simulink library "engine_T2_lib"  (Simulink 7.2)
settings: Solver=ode45  SolverMode=SingleTasking  StartTime=0.0  StopTime=10.0  RelTol=1e-3
undefined symbols (not defined in the file or in its folder): engl_ang, engr_ang, LengON, LinearizeModeOn, RengON, TrimModeOn
libraries: aeroutilslib x4, engine_JetCatP70_lib x4, simulink x3, Cross_Product_3D_lib x2
settings Model: Creator=amurch  LastModifiedBy=E183308

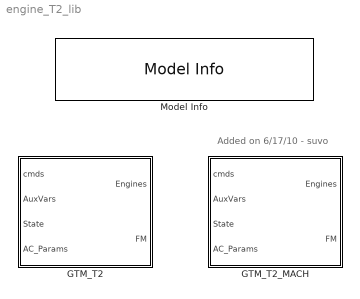
== system engine_T2_lib ==
  note: Added on 6/17/10 - suvo
  GTM_T2 : Subsystem
  GTM_T2_MACH : Subsystem
  Model Info : simulink/Model-Wide Utilities/Model Info  SystemSampleTime=-1  InitialBlockCM=None  BlockCM=None  Frame=on  DisplayStringWithTags=|  HorizontalTextAlignment=Center  LeftAlignmentValue=0.5  SourceBlockDiagram=engine_T2_lib  TagMaxNumber=20
      | GTM T2 Engine Library
      | 
      | Model Version: %<ModelVersion>
      | Last modifed by %<LastModifiedBy> on %<LastModificationDate>

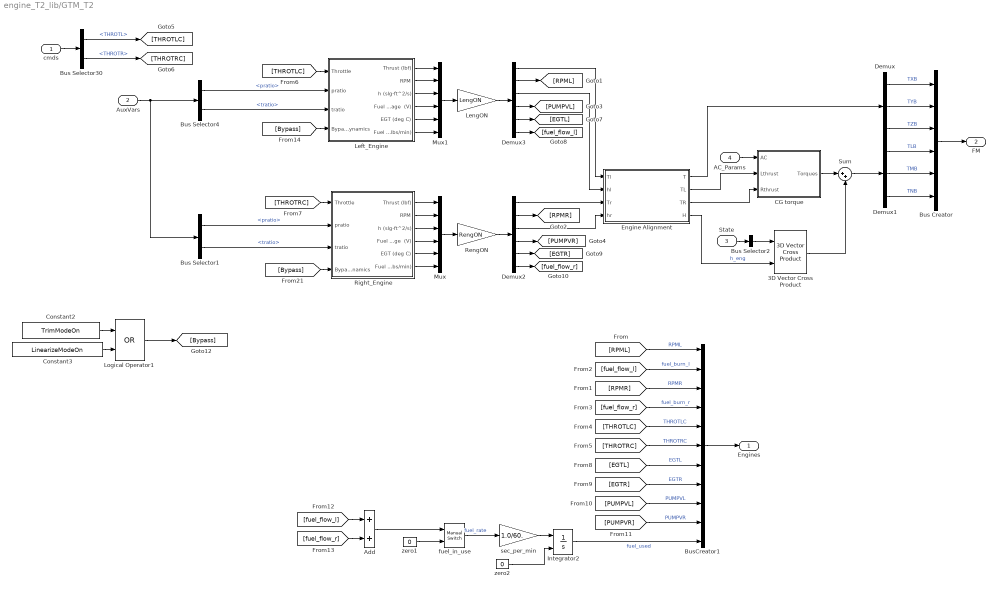
== system engine_T2_lib/GTM_T2 ==
  cmds : Inport  OutDataType=sfix(16)  OutScaling=2^0
  AuxVars : Inport  Port=2  OutDataType=sfix(16)  OutScaling=2^0
  State : Inport  Port=3  OutDataType=sfix(16)  OutScaling=2^0
  AC_Params : Inport  Port=4  OutDataType=sfix(16)  OutScaling=2^0
  3D Vector Cross Product : Cross_Product_3D_lib/3D Vector Cross Product  SystemSampleTime=-1
  Add : Sum  OutDataType=sfix(16)  OutScaling=2^-10
  Bus Creator : BusCreator  Inputs=6
  Bus Selector1 : BusSelector  OutputSignals=pratio,tratio
  Bus Selector2 : BusSelector  OutputSignals=pb,qb,rb  OutputAsBus=on
  Bus Selector30 : BusSelector  OutputSignals=THROTL,THROTR
  Bus Selector4 : BusSelector  OutputSignals=pratio,tratio
  BusCreator1 : BusCreator  Inputs=11
  CG torque : Subsystem
  Constant2 : Constant  Value=TrimModeOn  OutDataType=sfix(16)  OutScaling=2^0
  Constant3 : Constant  Value=LinearizeModeOn  OutDataType=sfix(16)  OutScaling=2^0
  Demux : Demux  Outputs=3
  Demux1 : Demux  Outputs=3
  Demux2 : Demux  Outputs=6
  Demux3 : Demux  Outputs=6
  Engine Alignment : Stateflow chart
  Integrator2 : Integrator  InitialConditionSource=external
  Left_Engine : Subsystem  BlockChoice=Jetcat P70
      settings: AttributesFormatString=%<BlockChoice>  TemplateBlock=enginelib/Engine Model  MemberBlocks=AMT-180,AMT-280,Blank,Jetcat P120SE,Jetcat P70
  LengON : Gain  Gain=LengON  ParameterDataType=sfix(16)  ParameterScaling=2^0  OutDataType=sfix(16)  OutScaling=2^0  SaturateOnIntegerOverflow=on  OutDataTypeStr=Inherit: Same as input  ParamDataTypeStr=Inherit: Same as input
  Logical Operator1 : Logic  Operator=OR  AllPortsSameDT=off  OutDataTypeMode=boolean  OutDataTypeStr=boolean
  Mux : Mux  Inputs=6
  Mux1 : Mux  Inputs=6
  RengON : Gain  Gain=RengON  ParameterDataType=sfix(16)  ParameterScaling=2^0  OutDataType=sfix(16)  OutScaling=2^0  SaturateOnIntegerOverflow=on  OutDataTypeStr=Inherit: Same as input  ParamDataTypeStr=Inherit: Same as input
  Right_Engine : Subsystem  BlockChoice=Jetcat P70
      settings: AttributesFormatString=%<BlockChoice>  TemplateBlock=enginelib/Engine Model  MemberBlocks=AMT-180,AMT-280,Blank,Jetcat P120SE,Jetcat P70
  Sum : Sum  Inputs=|++  OutDataType=sfix(16)  OutScaling=2^0
  fuel_in_use : simulink/Signal Routing/Manual Switch  SystemSampleTime=-1  sw=0  action=0  varsize=off
  sec_per_min : Gain  Gain=1.0/60.  ParameterDataType=sfix(16)  ParameterScaling=2^0  OutDataType=sfix(16)  OutScaling=2^0  SaturateOnIntegerOverflow=on  OutDataTypeStr=Inherit: Same as input  ParamDataTypeStr=Inherit: Same as input
  zero1 : Constant  Value=0  OutDataType=sfix(16)  OutScaling=2^0
  zero2 : Constant  Value=0  OutDataType=sfix(16)  OutScaling=2^0
  Engines : Outport  OutDataType=sfix(16)  OutScaling=2^0
  FM : Outport  Port=2  PortDimensions=6  OutDataType=sfix(16)  OutScaling=2^0
  wires:
  cmds/1 -> Bus Selector30/1
  Demux/2 -> Bus Creator/2  "TYB"
  State/1 -> Bus Selector2/1
  Bus Selector2/1 -> 3D Vector Cross Product/1
  Demux/3 -> Bus Creator/3  "TZB"
  Bus Selector1/1 -> Right_Engine/2(pratio)  "<pratio>"
  Bus Selector1/2 -> Right_Engine/3(tratio)  "<tratio>"
  AuxVars/1 -> Bus Selector1/1, Bus Selector4/1
  AC_Params/1 -> CG torque/1(AC)
  Bus Creator/1 -> FM/1
  Bus Selector30/1 -> [THROTLC]  "<THROTL>"
  Bus Selector30/2 -> [THROTRC]  "<THROTR>"
  [THROTLC] -> Left_Engine/1(Throttle)
  [THROTRC] -> Right_Engine/1(Throttle)
  [THROTRC] -> BusCreator1/6  "THROTRC"
  [THROTLC] -> BusCreator1/5  "THROTLC"
  [fuel_flow_r] -> BusCreator1/4  "fuel_burn_r"
  [fuel_flow_l] -> BusCreator1/2  "fuel_burn_l"
  [RPMR] -> BusCreator1/3  "RPMR"
  [RPML] -> BusCreator1/1  "RPML"
  BusCreator1/1 -> Engines/1
  [EGTL] -> BusCreator1/7  "EGTL"
  [EGTR] -> BusCreator1/8  "EGTR"
  [PUMPVL] -> BusCreator1/9  "PUMPVL"
  [PUMPVR] -> BusCreator1/10  "PUMPVR"
  sec_per_min/1 -> Integrator2/1
  fuel_in_use/1 -> sec_per_min/1  "fuel_rate"
  Integrator2/1 -> BusCreator1/11  "fuel_used"
  zero2/1 -> Integrator2/2
  [fuel_flow_l] -> Add/1
  [fuel_flow_r] -> Add/2
  zero1/1 -> fuel_in_use/2
  Add/1 -> fuel_in_use/1
  Bus Selector4/1 -> Left_Engine/2(pratio)  "<pratio>"
  Bus Selector4/2 -> Left_Engine/3(tratio)  "<tratio>"
  [Bypass] -> Left_Engine/4(BypassDynamics)
  [Bypass] -> Right_Engine/4(BypassDynamics)
  Demux/1 -> Bus Creator/1  "TXB"
  Engine Alignment/4(H) -> 3D Vector Cross Product/2  "h_eng"
  Engine Alignment/1(T) -> Demux/1
  Engine Alignment/2(TL) -> CG torque/2(Lthrust)
  Engine Alignment/3(TR) -> CG torque/3(Rthrust)
  CG torque/1(Torques) -> Sum/1
  3D Vector Cross Product/1 -> Sum/2
  Sum/1 -> Demux1/1
  Demux1/1 -> Bus Creator/4  "TLB"
  Demux1/2 -> Bus Creator/5  "TMB"
  Demux1/3 -> Bus Creator/6  "TNB"
  Right_Engine/1(Thrust (lbf)) -> Mux/1
  Right_Engine/2(RPM) -> Mux/2
  Right_Engine/3(h (slg-ft^2/s)) -> Mux/3
  Right_Engine/4(Fuel Pump Voltage  (V)) -> Mux/4
  Right_Engine/5(EGT (deg C)) -> Mux/5
  Right_Engine/6(Fuel Flow (lbs/min)) -> Mux/6
  Mux/1 -> RengON/1
  RengON/1 -> Demux2/1
  Demux2/1 -> Engine Alignment/3(Tr)
  Demux2/2 -> [RPMR]
  Demux2/3 -> Engine Alignment/4(hr)
  Demux2/4 -> [PUMPVR]
  Demux2/5 -> [EGTR]
  Demux2/6 -> [fuel_flow_r]
  Mux1/1 -> LengON/1
  LengON/1 -> Demux3/1
  Left_Engine/1(Thrust (lbf)) -> Mux1/1
  Left_Engine/2(RPM) -> Mux1/2
  Left_Engine/3(h (slg-ft^2/s)) -> Mux1/3
  Left_Engine/4(Fuel Pump Voltage  (V)) -> Mux1/4
  Left_Engine/5(EGT (deg C)) -> Mux1/5
  Left_Engine/6(Fuel Flow (lbs/min)) -> Mux1/6
  Demux3/1 -> Engine Alignment/1(Tl)
  Demux3/2 -> [RPML]
  Demux3/3 -> Engine Alignment/2(hl)
  Demux3/4 -> [PUMPVL]
  Demux3/5 -> [EGTL]
  Demux3/6 -> [fuel_flow_l]
  Constant3/1 -> Logical Operator1/2
  Constant2/1 -> Logical Operator1/1
  Logical Operator1/1 -> [Bypass]

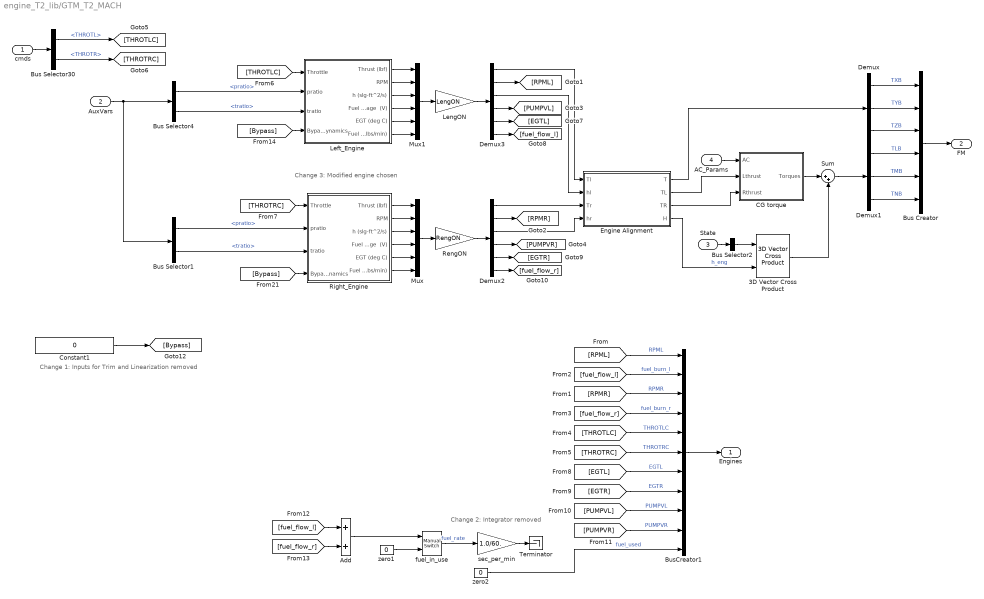
== system engine_T2_lib/GTM_T2_MACH ==
  note: Change 1: Inputs for Trim and Linearization removed
  note: Change 2: Integrator removed
  note: Change 3: Modified engine chosen
  cmds : Inport  OutDataType=sfix(16)  OutScaling=2^0
  AuxVars : Inport  Port=2  OutDataType=sfix(16)  OutScaling=2^0
  State : Inport  Port=3  OutDataType=sfix(16)  OutScaling=2^0
  AC_Params : Inport  Port=4  OutDataType=sfix(16)  OutScaling=2^0
  3D Vector Cross Product : Cross_Product_3D_lib/3D Vector Cross Product  SystemSampleTime=-1
  Add : Sum  OutDataType=sfix(16)  OutScaling=2^-10
  Bus Creator : BusCreator  Inputs=6
  Bus Selector1 : BusSelector  OutputSignals=pratio,tratio
  Bus Selector2 : BusSelector  OutputSignals=pb,qb,rb  OutputAsBus=on
  Bus Selector30 : BusSelector  OutputSignals=THROTL,THROTR
  Bus Selector4 : BusSelector  OutputSignals=pratio,tratio
  BusCreator1 : BusCreator  Inputs=11
  CG torque : Subsystem
  Constant1 : Constant  Value=0  OutDataType=sfix(16)  OutScaling=2^0
  Demux : Demux  Outputs=3
  Demux1 : Demux  Outputs=3
  Demux2 : Demux  Outputs=6
  Demux3 : Demux  Outputs=6
  Engine Alignment : Stateflow chart
  Left_Engine : Subsystem  BlockChoice=Jetcat P70_MACH
      settings: AttributesFormatString=%<BlockChoice>  TemplateBlock=enginelib/Engine Model  MemberBlocks=AMT-180,AMT-280,Blank,Jetcat P120SE,Jetcat P70,Jetcat P70_MACH
  LengON : Gain  Gain=LengON  ParameterDataType=sfix(16)  ParameterScaling=2^0  OutDataType=sfix(16)  OutScaling=2^0  SaturateOnIntegerOverflow=on  OutDataTypeStr=Inherit: Same as input  ParamDataTypeStr=Inherit: Same as input
  Mux : Mux  Inputs=6
  Mux1 : Mux  Inputs=6
  RengON : Gain  Gain=RengON  ParameterDataType=sfix(16)  ParameterScaling=2^0  OutDataType=sfix(16)  OutScaling=2^0  SaturateOnIntegerOverflow=on  OutDataTypeStr=Inherit: Same as input  ParamDataTypeStr=Inherit: Same as input
  Right_Engine : Subsystem  BlockChoice=Jetcat P70_MACH
      settings: AttributesFormatString=%<BlockChoice>  TemplateBlock=enginelib/Engine Model  MemberBlocks=AMT-180,AMT-280,Blank,Jetcat P120SE,Jetcat P70,Jetcat P70_MACH
  Sum : Sum  Inputs=|++  OutDataType=sfix(16)  OutScaling=2^0
  Terminator : Terminator
  fuel_in_use : simulink/Signal Routing/Manual Switch  SystemSampleTime=-1  sw=0  action=0  varsize=off
  sec_per_min : Gain  Gain=1.0/60.  ParameterDataType=sfix(16)  ParameterScaling=2^0  OutDataType=sfix(16)  OutScaling=2^0  SaturateOnIntegerOverflow=on  OutDataTypeStr=Inherit: Same as input  ParamDataTypeStr=Inherit: Same as input
  zero1 : Constant  Value=0  OutDataType=sfix(16)  OutScaling=2^0
  zero2 : Constant  Value=0  OutDataType=sfix(16)  OutScaling=2^0
  Engines : Outport  OutDataType=sfix(16)  OutScaling=2^0
  FM : Outport  Port=2  PortDimensions=6  OutDataType=sfix(16)  OutScaling=2^0
  wires:
  Constant1/1 -> [Bypass]
  Demux3/6 -> [fuel_flow_l]
  Demux3/5 -> [EGTL]
  Demux3/4 -> [PUMPVL]
  Demux3/3 -> Engine Alignment/2(hl)
  Demux3/2 -> [RPML]
  Demux3/1 -> Engine Alignment/1(Tl)
  Left_Engine/6(Fuel Flow (lbs/min)) -> Mux1/6
  Left_Engine/5(EGT (deg C)) -> Mux1/5
  Left_Engine/4(Fuel Pump Voltage  (V)) -> Mux1/4
  Left_Engine/3(h (slg-ft^2/s)) -> Mux1/3
  Left_Engine/2(RPM) -> Mux1/2
  Left_Engine/1(Thrust (lbf)) -> Mux1/1
  LengON/1 -> Demux3/1
  Mux1/1 -> LengON/1
  Demux2/6 -> [fuel_flow_r]
  Demux2/5 -> [EGTR]
  Demux2/4 -> [PUMPVR]
  Demux2/3 -> Engine Alignment/4(hr)
  Demux2/2 -> [RPMR]
  Demux2/1 -> Engine Alignment/3(Tr)
  RengON/1 -> Demux2/1
  Mux/1 -> RengON/1
  Right_Engine/6(Fuel Flow (lbs/min)) -> Mux/6
  Right_Engine/5(EGT (deg C)) -> Mux/5
  Right_Engine/4(Fuel Pump Voltage  (V)) -> Mux/4
  Right_Engine/3(h (slg-ft^2/s)) -> Mux/3
  Right_Engine/2(RPM) -> Mux/2
  Right_Engine/1(Thrust (lbf)) -> Mux/1
  Demux1/3 -> Bus Creator/6  "TNB"
  Demux1/2 -> Bus Creator/5  "TMB"
  Demux1/1 -> Bus Creator/4  "TLB"
  Sum/1 -> Demux1/1
  3D Vector Cross Product/1 -> Sum/2
  CG torque/1(Torques) -> Sum/1
  Engine Alignment/3(TR) -> CG torque/3(Rthrust)
  Engine Alignment/2(TL) -> CG torque/2(Lthrust)
  Engine Alignment/1(T) -> Demux/1
  Engine Alignment/4(H) -> 3D Vector Cross Product/2  "h_eng"
  Demux/1 -> Bus Creator/1  "TXB"
  [Bypass] -> Right_Engine/4(BypassDynamics)
  [Bypass] -> Left_Engine/4(BypassDynamics)
  Bus Selector4/2 -> Left_Engine/3(tratio)  "<tratio>"
  Bus Selector4/1 -> Left_Engine/2(pratio)  "<pratio>"
  Add/1 -> fuel_in_use/1
  zero1/1 -> fuel_in_use/2
  [fuel_flow_r] -> Add/2
  [fuel_flow_l] -> Add/1
  zero2/1 -> BusCreator1/11  "fuel_used"
  fuel_in_use/1 -> sec_per_min/1  "fuel_rate"
  sec_per_min/1 -> Terminator/1
  [PUMPVR] -> BusCreator1/10  "PUMPVR"
  [PUMPVL] -> BusCreator1/9  "PUMPVL"
  [EGTR] -> BusCreator1/8  "EGTR"
  [EGTL] -> BusCreator1/7  "EGTL"
  BusCreator1/1 -> Engines/1
  [RPML] -> BusCreator1/1  "RPML"
  [RPMR] -> BusCreator1/3  "RPMR"
  [fuel_flow_l] -> BusCreator1/2  "fuel_burn_l"
  [fuel_flow_r] -> BusCreator1/4  "fuel_burn_r"
  [THROTLC] -> BusCreator1/5  "THROTLC"
  [THROTRC] -> BusCreator1/6  "THROTRC"
  [THROTRC] -> Right_Engine/1(Throttle)
  [THROTLC] -> Left_Engine/1(Throttle)
  Bus Selector30/2 -> [THROTRC]  "<THROTR>"
  Bus Selector30/1 -> [THROTLC]  "<THROTL>"
  Bus Creator/1 -> FM/1
  AC_Params/1 -> CG torque/1(AC)
  AuxVars/1 -> Bus Selector4/1, Bus Selector1/1
  Bus Selector1/2 -> Right_Engine/3(tratio)  "<tratio>"
  Bus Selector1/1 -> Right_Engine/2(pratio)  "<pratio>"
  Demux/3 -> Bus Creator/3  "TZB"
  Bus Selector2/1 -> 3D Vector Cross Product/1
  State/1 -> Bus Selector2/1
  Demux/2 -> Bus Creator/2  "TYB"
  cmds/1 -> Bus Selector30/1

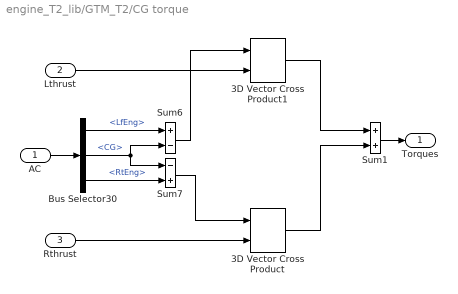
== system engine_T2_lib/GTM_T2/CG torque ==
  AC : Inport  OutDataType=sfix(16)  OutScaling=2^0
  Lthrust : Inport  Port=2  OutDataType=sfix(16)  OutScaling=2^0
  Rthrust : Inport  Port=3  OutDataType=sfix(16)  OutScaling=2^0
  3D Vector Cross Product : aeroutilslib/3D Vector Cross Product  SystemSampleTime=-1
  3D Vector Cross Product1 : aeroutilslib/3D Vector Cross Product  SystemSampleTime=-1
  Bus Selector30 : BusSelector  OutputSignals=LfEng,CG,RtEng
  Sum1 : Sum  OutDataType=sfix(16)  OutScaling=2^0  SaturateOnIntegerOverflow=on  InputSameDT=on  OutDataTypeStr=Inherit: Same as first input
  Sum6 : Sum  Inputs=+-  OutDataType=sfix(16)  OutScaling=2^0  SaturateOnIntegerOverflow=on  InputSameDT=on  OutDataTypeStr=Inherit: Same as first input
  Sum7 : Sum  Inputs=-+  OutDataType=sfix(16)  OutScaling=2^0  SaturateOnIntegerOverflow=on  InputSameDT=on  OutDataTypeStr=Inherit: Same as first input
  Torques : Outport  OutDataType=sfix(16)  OutScaling=2^0
  wires:
  AC/1 -> Bus Selector30/1
  Bus Selector30/2 -> Sum7/1, Sum6/2  "<CG>"
  Lthrust/1 -> 3D Vector Cross Product1/2
  Rthrust/1 -> 3D Vector Cross Product/2
  Sum7/1 -> 3D Vector Cross Product/1
  Sum6/1 -> 3D Vector Cross Product1/1
  3D Vector Cross Product1/1 -> Sum1/1
  3D Vector Cross Product/1 -> Sum1/2
  Sum1/1 -> Torques/1
  Bus Selector30/3 -> Sum7/2  "<RtEng>"
  Bus Selector30/1 -> Sum6/1  "<LfEng>"

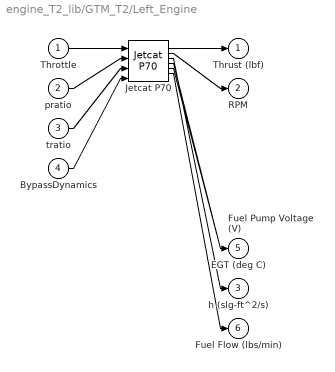
== system engine_T2_lib/GTM_T2/Left_Engine ==
  Throttle : Inport  OutDataType=sfix(16)  OutScaling=2^0
  pratio : Inport  Port=2  OutDataType=sfix(16)  OutScaling=2^0
  tratio : Inport  Port=3  OutDataType=sfix(16)  OutScaling=2^0
  BypassDynamics : Inport  Port=4  OutDataType=sfix(16)  OutScaling=2^0
  Jetcat P70 : engine_JetCatP70_lib/Jetcat P70  SystemSampleTime=-1
  Thrust (lbf) : Outport  OutDataType=sfix(16)  OutScaling=2^0
  RPM : Outport  Port=2  OutDataType=sfix(16)  OutScaling=2^0
  h (slg-ft^2/s) : Outport  Port=3  OutDataType=sfix(16)  OutScaling=2^0
  Fuel Pump Voltage  (V) : Outport  Port=4  OutDataType=sfix(16)  OutScaling=2^0
  EGT (deg C) : Outport  Port=5  OutDataType=sfix(16)  OutScaling=2^0
  Fuel Flow (lbs/min) : Outport  Port=6  OutDataType=sfix(16)  OutScaling=2^0
  wires:
  Throttle/1 -> Jetcat P70/1
  pratio/1 -> Jetcat P70/2
  tratio/1 -> Jetcat P70/3
  BypassDynamics/1 -> Jetcat P70/4
  Jetcat P70/1 -> Thrust (lbf)/1
  Jetcat P70/2 -> RPM/1
  Jetcat P70/3 -> h (slg-ft^2/s)/1
  Jetcat P70/4 -> Fuel Pump Voltage  (V)/1
  Jetcat P70/5 -> EGT (deg C)/1
  Jetcat P70/6 -> Fuel Flow (lbs/min)/1

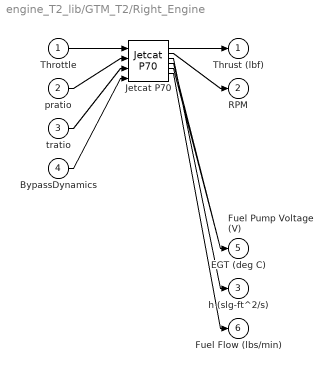
== system engine_T2_lib/GTM_T2/Right_Engine ==
  Throttle : Inport  OutDataType=sfix(16)  OutScaling=2^0
  pratio : Inport  Port=2  OutDataType=sfix(16)  OutScaling=2^0
  tratio : Inport  Port=3  OutDataType=sfix(16)  OutScaling=2^0
  BypassDynamics : Inport  Port=4  OutDataType=sfix(16)  OutScaling=2^0
  Jetcat P70 : engine_JetCatP70_lib/Jetcat P70  SystemSampleTime=-1
  Thrust (lbf) : Outport  OutDataType=sfix(16)  OutScaling=2^0
  RPM : Outport  Port=2  OutDataType=sfix(16)  OutScaling=2^0
  h (slg-ft^2/s) : Outport  Port=3  OutDataType=sfix(16)  OutScaling=2^0
  Fuel Pump Voltage  (V) : Outport  Port=4  OutDataType=sfix(16)  OutScaling=2^0
  EGT (deg C) : Outport  Port=5  OutDataType=sfix(16)  OutScaling=2^0
  Fuel Flow (lbs/min) : Outport  Port=6  OutDataType=sfix(16)  OutScaling=2^0
  wires:
  Throttle/1 -> Jetcat P70/1
  pratio/1 -> Jetcat P70/2
  tratio/1 -> Jetcat P70/3
  BypassDynamics/1 -> Jetcat P70/4
  Jetcat P70/1 -> Thrust (lbf)/1
  Jetcat P70/2 -> RPM/1
  Jetcat P70/3 -> h (slg-ft^2/s)/1
  Jetcat P70/4 -> Fuel Pump Voltage  (V)/1
  Jetcat P70/5 -> EGT (deg C)/1
  Jetcat P70/6 -> Fuel Flow (lbs/min)/1

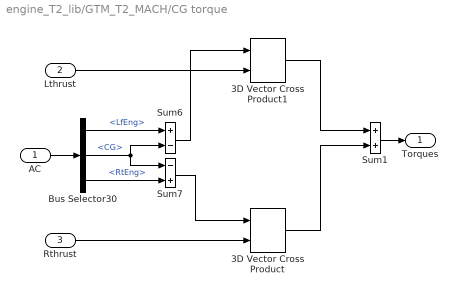
== system engine_T2_lib/GTM_T2_MACH/CG torque ==
  AC : Inport  OutDataType=sfix(16)  OutScaling=2^0
  Lthrust : Inport  Port=2  OutDataType=sfix(16)  OutScaling=2^0
  Rthrust : Inport  Port=3  OutDataType=sfix(16)  OutScaling=2^0
  3D Vector Cross Product : aeroutilslib/3D Vector Cross Product  SystemSampleTime=-1
  3D Vector Cross Product1 : aeroutilslib/3D Vector Cross Product  SystemSampleTime=-1
  Bus Selector30 : BusSelector  OutputSignals=LfEng,CG,RtEng
  Sum1 : Sum  OutDataType=sfix(16)  OutScaling=2^0  SaturateOnIntegerOverflow=on  InputSameDT=on  OutDataTypeStr=Inherit: Same as first input
  Sum6 : Sum  Inputs=+-  OutDataType=sfix(16)  OutScaling=2^0  SaturateOnIntegerOverflow=on  InputSameDT=on  OutDataTypeStr=Inherit: Same as first input
  Sum7 : Sum  Inputs=-+  OutDataType=sfix(16)  OutScaling=2^0  SaturateOnIntegerOverflow=on  InputSameDT=on  OutDataTypeStr=Inherit: Same as first input
  Torques : Outport  OutDataType=sfix(16)  OutScaling=2^0
  wires:
  Bus Selector30/1 -> Sum6/1  "<LfEng>"
  Bus Selector30/3 -> Sum7/2  "<RtEng>"
  Sum1/1 -> Torques/1
  3D Vector Cross Product/1 -> Sum1/2
  3D Vector Cross Product1/1 -> Sum1/1
  Sum6/1 -> 3D Vector Cross Product1/1
  Sum7/1 -> 3D Vector Cross Product/1
  Rthrust/1 -> 3D Vector Cross Product/2
  Lthrust/1 -> 3D Vector Cross Product1/2
  Bus Selector30/2 -> Sum6/2, Sum7/1  "<CG>"
  AC/1 -> Bus Selector30/1

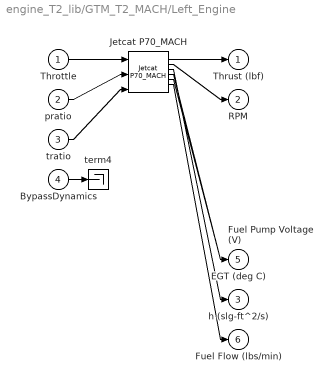
== system engine_T2_lib/GTM_T2_MACH/Left_Engine ==
  Throttle : Inport  OutDataType=sfix(16)  OutScaling=2^0
  pratio : Inport  Port=2  OutDataType=sfix(16)  OutScaling=2^0
  tratio : Inport  Port=3  OutDataType=sfix(16)  OutScaling=2^0
  BypassDynamics : Inport  Port=4  OutDataType=sfix(16)  OutScaling=2^0
  Jetcat P70_MACH : engine_JetCatP70_lib/Jetcat P70_MACH  SystemSampleTime=-1
  term4 : Terminator
  Thrust (lbf) : Outport  OutDataType=sfix(16)  OutScaling=2^0
  RPM : Outport  Port=2  OutDataType=sfix(16)  OutScaling=2^0
  h (slg-ft^2/s) : Outport  Port=3  OutDataType=sfix(16)  OutScaling=2^0
  Fuel Pump Voltage  (V) : Outport  Port=4  OutDataType=sfix(16)  OutScaling=2^0
  EGT (deg C) : Outport  Port=5  OutDataType=sfix(16)  OutScaling=2^0
  Fuel Flow (lbs/min) : Outport  Port=6  OutDataType=sfix(16)  OutScaling=2^0
  wires:
  Throttle/1 -> Jetcat P70_MACH/1
  pratio/1 -> Jetcat P70_MACH/2
  tratio/1 -> Jetcat P70_MACH/3
  Jetcat P70_MACH/1 -> Thrust (lbf)/1
  Jetcat P70_MACH/2 -> RPM/1
  Jetcat P70_MACH/3 -> h (slg-ft^2/s)/1
  Jetcat P70_MACH/4 -> Fuel Pump Voltage  (V)/1
  Jetcat P70_MACH/5 -> EGT (deg C)/1
  Jetcat P70_MACH/6 -> Fuel Flow (lbs/min)/1
  BypassDynamics/1 -> term4/1

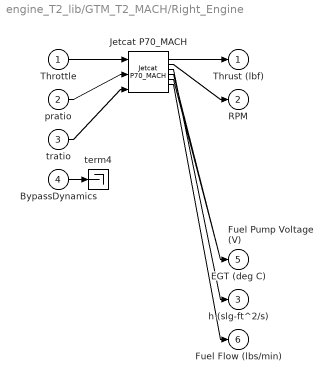
== system engine_T2_lib/GTM_T2_MACH/Right_Engine ==
  Throttle : Inport  OutDataType=sfix(16)  OutScaling=2^0
  pratio : Inport  Port=2  OutDataType=sfix(16)  OutScaling=2^0
  tratio : Inport  Port=3  OutDataType=sfix(16)  OutScaling=2^0
  BypassDynamics : Inport  Port=4  OutDataType=sfix(16)  OutScaling=2^0
  Jetcat P70_MACH : engine_JetCatP70_lib/Jetcat P70_MACH  SystemSampleTime=-1
  term4 : Terminator
  Thrust (lbf) : Outport  OutDataType=sfix(16)  OutScaling=2^0
  RPM : Outport  Port=2  OutDataType=sfix(16)  OutScaling=2^0
  h (slg-ft^2/s) : Outport  Port=3  OutDataType=sfix(16)  OutScaling=2^0
  Fuel Pump Voltage  (V) : Outport  Port=4  OutDataType=sfix(16)  OutScaling=2^0
  EGT (deg C) : Outport  Port=5  OutDataType=sfix(16)  OutScaling=2^0
  Fuel Flow (lbs/min) : Outport  Port=6  OutDataType=sfix(16)  OutScaling=2^0
  wires:
  Throttle/1 -> Jetcat P70_MACH/1
  pratio/1 -> Jetcat P70_MACH/2
  tratio/1 -> Jetcat P70_MACH/3
  Jetcat P70_MACH/1 -> Thrust (lbf)/1
  Jetcat P70_MACH/2 -> RPM/1
  Jetcat P70_MACH/3 -> h (slg-ft^2/s)/1
  Jetcat P70_MACH/4 -> Fuel Pump Voltage  (V)/1
  Jetcat P70_MACH/5 -> EGT (deg C)/1
  Jetcat P70_MACH/6 -> Fuel Flow (lbs/min)/1
  BypassDynamics/1 -> term4/1

== matlab function GTM_T2_MACH/Engine Alignment ==
  data: T output double; Tl input double; hl input double; Tr input double; hr input double; TL output double; engl_ang parameter double; engr_ang parameter double; TR output double; H output double
function [T,TL,TR,H] = eng_angles(Tl,hl,Tr,hr,engl_ang,engr_ang)
% This block supports an embeddable subset of the MATLAB language.
% See the help menu for details. 

% Using the engine alignment angles (set in AC_params_T2.m), compute the 
% off-axis thrust and angular momentum terms.

TL = Tl*[cosd(engl_ang(2))*cosd(engl_ang(3));...
         sind(engl_ang(3));...
         -sind(engl_ang(2))*cosd(engl_ang(3))];
TR = Tr*[cosd(engr_ang(2))*cosd(engr_ang(3));...
         sind(engr_ang(3));...
         -sind(engr_ang(2))*cosd(engr_ang(3))];  
T = TL+TR;

H = hl*[cosd(engl_ang(2))*cosd(engl_ang(3));...
         sind(engl_ang(3));...
         -sind(engl_ang(2))*cosd(engl_ang(3))] + ...
         hr*[cosd(engr_ang(2))*cosd(engr_ang(3));...
         sind(engr_ang(3));...
         -sind(engr_ang(2))*cosd(engr_ang(3))];

== matlab function GTM_T2/Engine Alignment ==
  data: T output double; Tl input double; hl input double; Tr input double; hr input double; TL output double; engl_ang parameter double; engr_ang parameter double; TR output double; H output double
function [T,TL,TR,H] = eng_angles(Tl,hl,Tr,hr,engl_ang,engr_ang)
% This block supports an embeddable subset of the MATLAB language.
% See the help menu for details. 

% Using the engine alignment angles (set in AC_params_T2.m), compute the 
% off-axis thrust and angular momentum terms.

TL = Tl*[cosd(engl_ang(2))*cosd(engl_ang(3));...
         sind(engl_ang(3));...
         -sind(engl_ang(2))*cosd(engl_ang(3))];
TR = Tr*[cosd(engr_ang(2))*cosd(engr_ang(3));...
         sind(engr_ang(3));...
         -sind(engr_ang(2))*cosd(engr_ang(3))];  
T = TL+TR;

H = hl*[cosd(engl_ang(2))*cosd(engl_ang(3));...
         sind(engl_ang(3));...
         -sind(engl_ang(2))*cosd(engl_ang(3))] + ...
         hr*[cosd(engr_ang(2))*cosd(engr_ang(3));...
         sind(engr_ang(3));...
         -sind(engr_ang(2))*cosd(engr_ang(3))];
